simulink model "simple_PD"  (R2021a)
settings: Solver=FixedStepAuto  StartTime=0.0  StopTime=inf  FixedStep=.001  RelTol=1e-3  EnableMultiTasking=on
model workspace (MAT data in the model file):
  SL_ROS_VariableLengthArrays_MaxSizes.CommonInfo.ArrayTruncateAction = 'EmitWarning'
  SL_ROS_VariableLengthArrays_MaxSizes.MsgTypeMap = containers.Map
  SL_ROS_VariableLengthArrays_MaxSizes.MsgTypeMap.serialization.keys = {'ambf_walker/DesiredJoints', 'sensor_msgs/JointState', 'std_msgs/Float32MultiArray'}
  SL_ROS_VariableLengthArrays_MaxSizes.MsgTypeMap.serialization.values{1}(1).PropertyName = 'Controller'
  SL_ROS_VariableLengthArrays_MaxSizes.MsgTypeMap.serialization.values{1}(1).DataType = 'uint8'
  SL_ROS_VariableLengthArrays_MaxSizes.MsgTypeMap.serialization.values{1}(1).MaxLength = 8
  SL_ROS_VariableLengthArrays_MaxSizes.MsgTypeMap.serialization.values{1}(2).PropertyName = 'Other'
  SL_ROS_VariableLengthArrays_MaxSizes.MsgTypeMap.serialization.values{1}(2).DataType = 'double'
  SL_ROS_VariableLengthArrays_MaxSizes.MsgTypeMap.serialization.values{1}(2).MaxLength = 7
  SL_ROS_VariableLengthArrays_MaxSizes.MsgTypeMap.serialization.values{1}(3).PropertyName = 'Q'
  SL_ROS_VariableLengthArrays_MaxSizes.MsgTypeMap.serialization.values{1}(3).DataType = 'double'
  SL_ROS_VariableLengthArrays_MaxSizes.MsgTypeMap.serialization.values{1}(3).MaxLength = 7
  SL_ROS_VariableLengthArrays_MaxSizes.MsgTypeMap.serialization.values{1}(4).PropertyName = 'Qd'
  SL_ROS_VariableLengthArrays_MaxSizes.MsgTypeMap.serialization.values{1}(4).DataType = 'double'
  SL_ROS_VariableLengthArrays_MaxSizes.MsgTypeMap.serialization.values{1}(4).MaxLength = 7
  SL_ROS_VariableLengthArrays_MaxSizes.MsgTypeMap.serialization.values{1}(5).PropertyName = 'Qdd'
  SL_ROS_VariableLengthArrays_MaxSizes.MsgTypeMap.serialization.values{1}(5).DataType = 'double'
  SL_ROS_VariableLengthArrays_MaxSizes.MsgTypeMap.serialization.values{1}(5).MaxLength = 7
  SL_ROS_VariableLengthArrays_MaxSizes.MsgTypeMap.serialization.values{2}(1).PropertyName = 'Effort'
  SL_ROS_VariableLengthArrays_MaxSizes.MsgTypeMap.serialization.values{2}(1).DataType = 'double'
  SL_ROS_VariableLengthArrays_MaxSizes.MsgTypeMap.serialization.values{2}(1).MaxLength = 7
  SL_ROS_VariableLengthArrays_MaxSizes.MsgTypeMap.serialization.values{2}(2).PropertyName = 'Name'
  SL_ROS_VariableLengthArrays_MaxSizes.MsgTypeMap.serialization.values{2}(2).DataType = 'std_msgs/String'
  SL_ROS_VariableLengthArrays_MaxSizes.MsgTypeMap.serialization.values{2}(2).MaxLength = 16
  SL_ROS_VariableLengthArrays_MaxSizes.MsgTypeMap.serialization.values{2}(3).PropertyName = 'Position'
  SL_ROS_VariableLengthArrays_MaxSizes.MsgTypeMap.serialization.values{2}(3).DataType = 'double'
  SL_ROS_VariableLengthArrays_MaxSizes.MsgTypeMap.serialization.values{2}(3).MaxLength = 7
  SL_ROS_VariableLengthArrays_MaxSizes.MsgTypeMap.serialization.values{2}(4).PropertyName = 'Velocity'
  SL_ROS_VariableLengthArrays_MaxSizes.MsgTypeMap.serialization.values{2}(4).DataType = 'double'
  SL_ROS_VariableLengthArrays_MaxSizes.MsgTypeMap.serialization.values{2}(4).MaxLength = 7
  SL_ROS_VariableLengthArrays_MaxSizes.MsgTypeMap.serialization.values{3}.PropertyName = 'Data'
  SL_ROS_VariableLengthArrays_MaxSizes.MsgTypeMap.serialization.values{3}.DataType = 'single'
  SL_ROS_VariableLengthArrays_MaxSizes.MsgTypeMap.serialization.values{3}.MaxLength = 7
  SL_ROS_VariableLengthArrays_MaxSizes.MsgTypeMap.serialization.uniformity = 0
  SL_ROS_VariableLengthArrays_MaxSizes.MsgTypeMap.serialization.keyType = 'char'
  SL_ROS_VariableLengthArrays_MaxSizes.MsgTypeMap.serialization.valueType = 'any'
values from neighbouring files (symbols this model uses):
  Dm1 = [Dm_hip, 0.0, 0.0, 0.0, 0.0, 0.0,0 ... (first row only)    [init_PD_Controller.m]
  Km1 = [Km_hip, 0.0, 0.0, 0.0, 0.0, 0.0,0 ... (first row only)    [init_PD_Controller.m]
undefined symbols (not defined in the file or in its folder): Effort, Header, l, mh, Position, Velocity
libraries: robotlib x13
settings Model: Creator=nathanielgoldfarb  LastModifiedBy=nathanielgoldfarb
settings OptimizationCC: StrengthReduction=on  PassReuseOutputArgsAs=Individual arguments  ZeroExternalMemoryAtStartup=off  ZeroInternalMemoryAtStartup=off  MaxStackSize=64  OptimizeBlockOrder=speed  OptimizationPriority=Speed  OptimizationCustomize=off  MultiThreadedLoops=on  EfficientTunableParamExpr=on
settings DebuggingCC: ParameterTunabilityLossMsg=error
settings HardwareCC: ProdBitPerPointer=32  ProdBitPerSizeT=32  ProdBitPerPtrDiffT=32  ProdLargestAtomicFloat=None  ProdIntDivRoundTo=Undefined  ProdEndianess=Unspecified  ProdWordSize=32  ProdHWDeviceType=Generic->Unspecified (assume 32-bit Generic)
settings SFSimCC: MATLABDynamicMemAlloc=off
settings RTWCC: SystemTargetFile=ert.tlc  HardwareBoard=Robot Operating System (ROS)  TLCOptions="-aInlineSetEventsForThisBaseRateFcn=TLC_FALSE -aSuppressMultiTaskScheduler=TLC_FALSE  -aRateBasedStepFcn=0"  TemplateMakefile=ert_default_tmf  Toolchain=Catkin  TargetLang=C++
settings CodeAppCC: ForceParamTrailComments=on  IgnoreCustomStorageClasses=off  OperatorAnnotations=on  SimulinkDataObjDesc=on  SFDataObjDesc=on  InsertBlockDesc=on

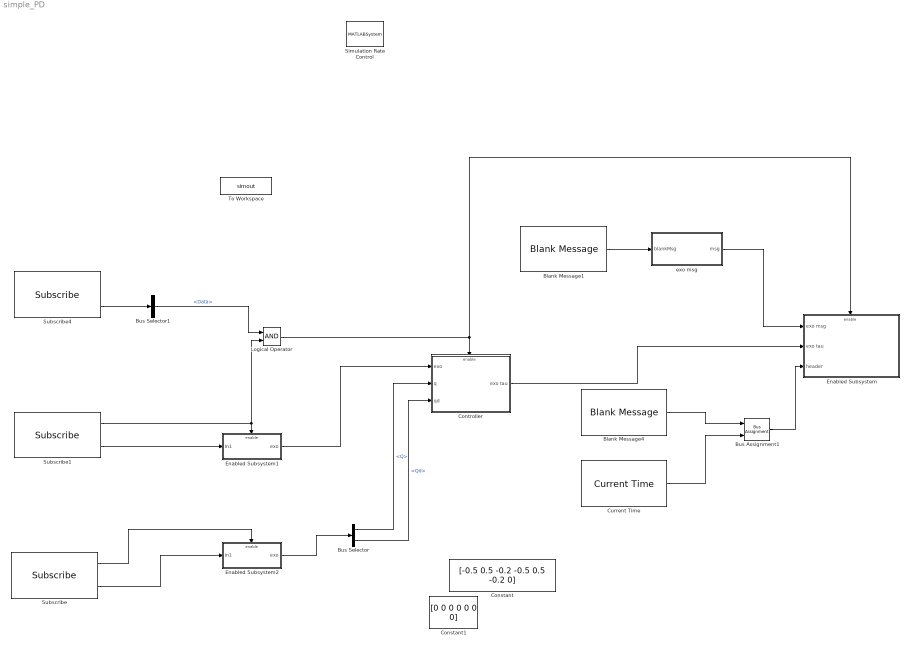
== system simple_PD ==
  Blank Message1 : robotlib/Blank Message  messageClass=Message  entityType=sensor_msgs/JointState  messageType=sensor_msgs/JointState  SampleTime=inf  legacyBusStruct=off
  Blank Message4 : robotlib/Blank Message  messageClass=Message  entityType=std_msgs/Header  messageType=std_msgs/Header  SampleTime=inf  legacyBusStruct=off
  Bus Assignment1 : BusAssignment  AssignedSignals=Stamp
  Bus Selector : BusSelector  OutputSignals=Q,Qd
  Bus Selector1 : BusSelector  OutputSignals=Data
  Constant : Constant  Value=[-0.5 0.5 -0.2 -0.5 0.5 -0.2 0]
  Constant1 : Constant  Value=[0 0 0 0 0 0 0]
  Controller : Subsystem  TreatAsAtomicUnit=on
  Current Time : robotlib/Current Time  OutputFormat=bus  SampleTime=-1  ModelName=simple_PD
      settings: SourceProductBaseCode=RR
  Enabled Subsystem : Subsystem  TreatAsAtomicUnit=on
  Enabled Subsystem1 : Subsystem  TreatAsAtomicUnit=on
  Enabled Subsystem2 : Subsystem  TreatAsAtomicUnit=on
  Logical Operator : Logic  AllPortsSameDT=off  OutDataTypeStr=boolean
  Simulation Rate Control : MATLABSystem  System=ExampleHelperSimulationRateControl  SampleTime=0.001
      mask Type: ExampleHelperSimulationRateControl
      mask Display:
      | disp('Rate Control');
      | port_label('output',1,'r');
  Subscribe : robotlib/Subscribe  topicSource=Select from ROS network  topic=/exosimulink_set_points  messageType=ambf_walker/DesiredJoints  SampleTime=-1  legacyBusStruct=off  messageQueueLength=1
  Subscribe1 : robotlib/Subscribe  topicSource=Select from ROS network  topic=/exo_jointstate  messageType=sensor_msgs/JointState  SampleTime=-1  legacyBusStruct=off  messageQueueLength=1
  Subscribe4 : robotlib/Subscribe  topicSource=Specify your own  topic=/start_sim  messageType=std_msgs/Bool  SampleTime=-1  legacyBusStruct=off  messageQueueLength=1
  To Workspace : ToWorkspace  VariableName=simout  SampleTime=-1
      settings: Save2DSignal=2-D array (concatenate along first dimension)
  exo msg : MATLAB Function  TreatAsAtomicUnit=on
  wires:
  Bus Assignment1/1 -> Enabled Subsystem/3(header)
  Blank Message1/1 -> exo msg/1(blankMsg)
  exo msg/1(msg) -> Enabled Subsystem/1(exo msg)
  Current Time/1 -> Bus Assignment1/2
  Blank Message4/1 -> Bus Assignment1/1
  Enabled Subsystem1/1(exo) -> Controller/1(exo)
  Subscribe4/2 -> Bus Selector1/1
  Subscribe1/2 -> Enabled Subsystem1/1(In1)
  Controller/1(exo tau) -> Enabled Subsystem/2(exo tau)
  Subscribe1/1 -> Enabled Subsystem1/Enable, Logical Operator/2
  Subscribe/2 -> Enabled Subsystem2/1(In1)
  Enabled Subsystem2/1(exo) -> Bus Selector/1
  Subscribe/1 -> Enabled Subsystem2/Enable
  Bus Selector1/1 -> Logical Operator/1  "<Data>"
  Logical Operator/1 -> Enabled Subsystem/Enable, Controller/Enable
  Bus Selector/1 -> Controller/2(q)  "<Q>"
  Bus Selector/2 -> Controller/3(qd)  "<Qd>"

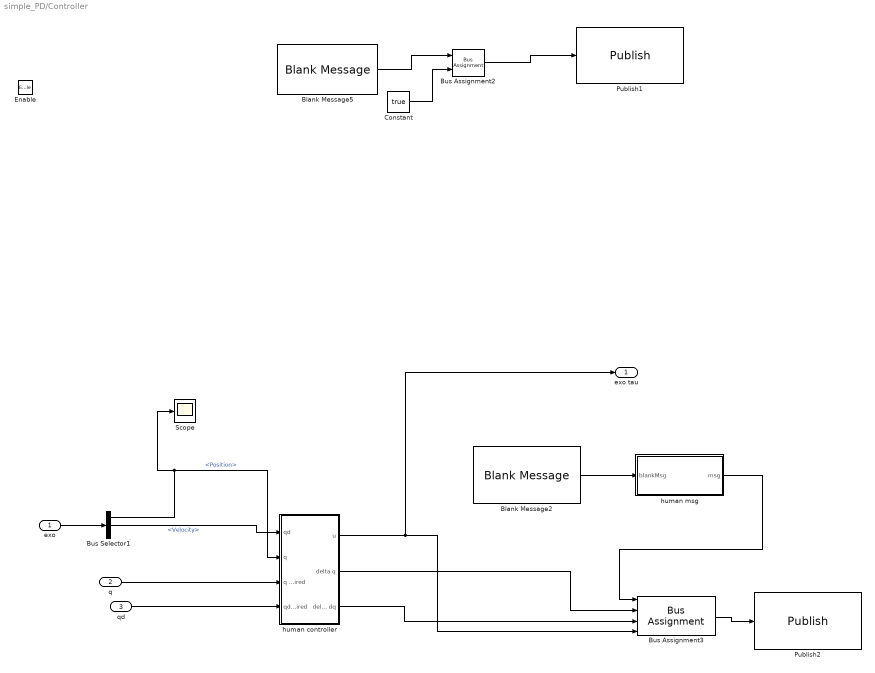
== system simple_PD/Controller ==
  exo : Inport
  q : Inport  Port=2
  qd : Inport  Port=3
  Enable : EnablePort
  Blank Message2 : robotlib/Blank Message  messageClass=Message  entityType=sensor_msgs/JointState  messageType=sensor_msgs/JointState  SampleTime=inf  legacyBusStruct=off
  Blank Message5 : robotlib/Blank Message  messageClass=Message  entityType=std_msgs/Bool  messageType=std_msgs/Bool  SampleTime=inf  legacyBusStruct=off
  Bus Assignment2 : BusAssignment  AssignedSignals=Data
  Bus Assignment3 : BusAssignment  AssignedSignals=Position,Velocity,Effort
  Bus Selector1 : BusSelector  OutputSignals=Position,Velocity,Effort
  Constant : Constant  Value=true  VectorParams1D=off
  Publish1 : robotlib/Publish  topicSource=Specify your own  topic=/my_topic  messageType=std_msgs/Bool  legacyBusStruct=off  messageQueueLength=1
  Publish2 : robotlib/Publish  topicSource=Specify your own  topic=addmittance  messageType=sensor_msgs/JointState  legacyBusStruct=off  messageQueueLength=1
  Scope : Scope
  human controller : Subsystem
  human msg : MATLAB Function  TreatAsAtomicUnit=on
  exo tau : Outport
  wires:
  q/1 -> human controller/3(q desired)
  qd/1 -> human controller/4(qd desired)
  Bus Selector1/1 -> human controller/2(q), Scope/1  "<Position>"
  exo/1 -> Bus Selector1/1
  Constant/1 -> Bus Assignment2/2
  Blank Message5/1 -> Bus Assignment2/1
  Bus Assignment2/1 -> Publish1/1
  Bus Assignment3/1 -> Publish2/1
  Blank Message2/1 -> human msg/1(blankMsg)
  human msg/1(msg) -> Bus Assignment3/1
  Bus Selector1/2 -> human controller/1(qd)  "<Velocity>"
  human controller/2(delta q) -> Bus Assignment3/2
  human controller/3(delta dq) -> Bus Assignment3/3
  human controller/1(u) -> exo tau/1, Bus Assignment3/4

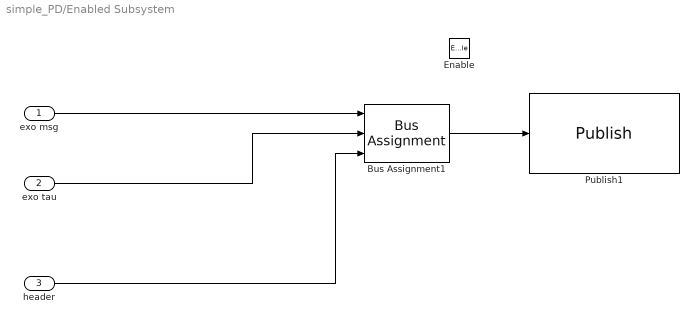
== system simple_PD/Enabled Subsystem ==
  exo msg : Inport
  exo tau : Inport  Port=2
  header : Inport  Port=3
  Enable : EnablePort
  Bus Assignment1 : BusAssignment  AssignedSignals=Effort,Header
  Publish1 : robotlib/Publish  topicSource=Select from ROS network  topic=/exo_simulink_torque  messageType=sensor_msgs/JointState  legacyBusStruct=off  messageQueueLength=1
  wires:
  exo tau/1 -> Bus Assignment1/2
  Bus Assignment1/1 -> Publish1/1
  exo msg/1 -> Bus Assignment1/1
  header/1 -> Bus Assignment1/3

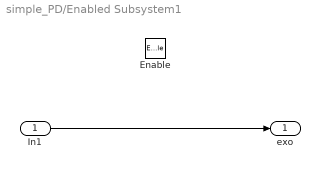
== system simple_PD/Enabled Subsystem1 ==
  In1 : Inport
  Enable : EnablePort
  exo : Outport
  wires:
  In1/1 -> exo/1

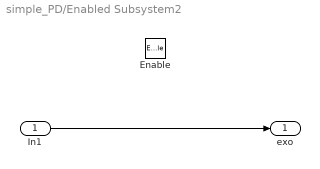
== system simple_PD/Enabled Subsystem2 ==
  In1 : Inport
  Enable : EnablePort
  exo : Outport
  wires:
  In1/1 -> exo/1

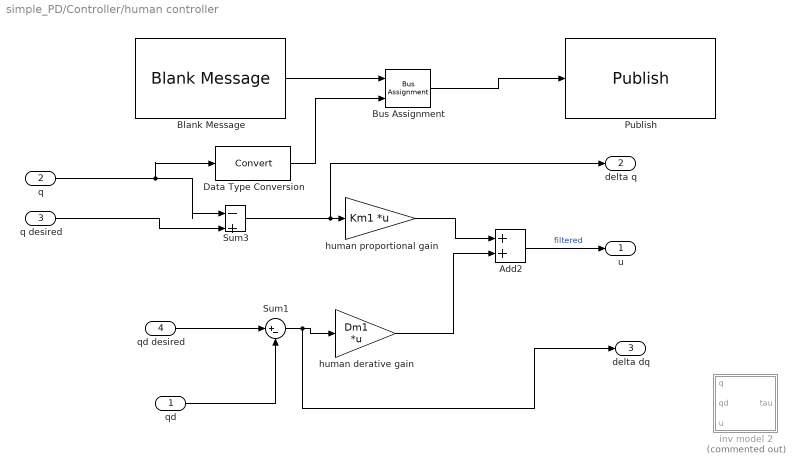
== system simple_PD/Controller/human controller ==
  qd : Inport
  q : Inport  Port=2
  q desired : Inport  Port=3
  qd desired : Inport  Port=4
  Add2 : Sum
  Blank Message : robotlib/Blank Message  messageClass=Message  entityType=std_msgs/Float32MultiArray  messageType=std_msgs/Float32MultiArray  SampleTime=inf  legacyBusStruct=off
  Bus Assignment : BusAssignment  AssignedSignals=Data
  Data Type Conversion : DataTypeConversion  RndMeth=Simplest
  Publish : robotlib/Publish  topicSource=Specify your own  topic=PD_error  messageType=std_msgs/Float32MultiArray  legacyBusStruct=off  messageQueueLength=1
  Sum1 : Sum  Inputs=|+-
  Sum3 : Sum  Inputs=|-+
  human derative gain : Gain  Gain=Dm1  Multiplication=Matrix(K*u)
  human proportional gain : Gain  Gain=Km1  Multiplication=Matrix(K*u)
  inv model 2 : Subsystem  Commented=on
  u : Outport
  delta q : Outport  Port=2
  delta dq : Outport  Port=3
  wires:
  Sum1/1 -> delta dq/1, human derative gain/1
  qd/1 -> Sum1/2
  Sum3/1 -> delta q/1, human proportional gain/1
  human derative gain/1 -> Add2/2
  q desired/1 -> Sum3/2
  human proportional gain/1 -> Add2/1
  qd desired/1 -> Sum1/1
  q/1 -> Data Type Conversion/1, Sum3/1
  Add2/1 -> u/1  "filtered"
  Blank Message/1 -> Bus Assignment/1
  Bus Assignment/1 -> Publish/1
  Data Type Conversion/1 -> Bus Assignment/2

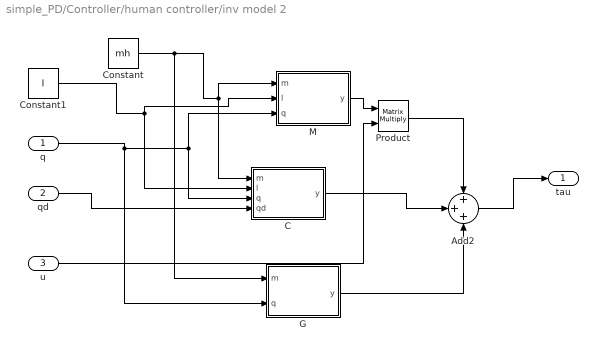
== system simple_PD/Controller/human controller/inv model 2 ==
  q : Inport
  qd : Inport  Port=2
  "u " : Inport  Port=3
  Add2 : Sum  Inputs=+++
  C : MATLAB Function  TreatAsAtomicUnit=on
  Constant : Constant  Value=mh
  Constant1 : Constant  Value=l
  G : MATLAB Function  TreatAsAtomicUnit=on
  M : MATLAB Function  TreatAsAtomicUnit=on
  Product : Product  Multiplication=Matrix(*)
  "tau " : Outport
  wires:
  Constant1/1 -> C/2(l), M/2(l)
  Constant/1 -> G/1(m), C/1(m), M/1(m)
  "u "/1 -> Product/2
  Product/1 -> Add2/1
  M/1(y) -> Product/1
  qd/1 -> C/4(qd)
  q/1 -> G/2(q), C/3(q), M/3(q)
  Add2/1 -> "tau "/1
  C/1(y) -> Add2/2
  G/1(y) -> Add2/3

== matlab function simple_PD/Controller/human controller/inv model 2/C ==
  data: m input; l input; q input; y output; qd input
function y = fcn(m, l, q, qd)



y = C(m, l, q, qd); % [m(2)*l(2)*qd(2)*qd(2)*sin(q(1)-q(2)); -m(2)*l(1)*qd(1)*qd(1)*sin(q(1)-q(2))];

== matlab function simple_PD/Controller/human controller/inv model 2/G ==
  data: m input; q input; y output
function y = fcn(m, q)
 y =  G(m,q);
end

== matlab function simple_PD/Controller/human controller/inv model 2/M ==
  data: m input; l input; q input; y output
function y = fcn(m, l, q)

y = M(m,l,q); % pinv([ (m(1)+m(2)) *l(1), m(2)*l(2)*cos(q(1)-q(2)); m(2)* l(1)*cos(q(1)-q(2)), m(2)*l(2)] );

end

== matlab function simple_PD/exo msg ==
  data: blankMsg input; msg output Bus: SL_Bus_simple_PD_sensor_msgs_JointState
function msg = stringArrayAssign(blankMsg)
% stringArrayAssign - Assign a string array in a ROS message
%
%  blankMsg (input): A bus for a 'sensor_msgs/JointState' message. This is 
%      used to initialize the output.
%  msg (output): A bus for a 'sensor_msgs/JointState' message message, with 
%      Name field set to a string array.
%
%   Copyright 2015 The MathWorks, Inc.

%#codegen

% Note: The datatype of 'msg' has been explicitly set to the appropriate 
% Simulink bus type ("SL_Bus_robotROSMessageUsageExample_sensor_msgs_JointState"). 
%
% If the model name is changed, the datatype needs to be changed as well:
%   1) Click "Edit Data" in the Editor toolstrip to open "Ports and Data Manager"
%   2) Select "msg". From the "Type" dropdown, select "--- Refresh data types ---"
%   3) Set datatype to "Bus: SL_Bus_<modelname>_sensor_msgs_JointState"

strArrayToAssign = {'LeftExoHip', 'LeftExoKnee', 'LeftExoAnkle', 'RightExoHip', 'RightExoKnee', 'RightExoAnkle', 'Crutches'};
msg = blankMsg;

% Set the number of strings in the string array.
% msg (sensor_msgs/JointState) includes the following fields
%           Name : array of std_msgs/String (string array)
%   Name_SL_Info : struct with fields CurrentLength, ReceivedLength
numStringsInArray = length(strArrayToAssign);
msg.Name_SL_Info.CurrentLength = uint32(numStringsInArray);
msg.Effort_SL_Info.CurrentLength = uint32(numStringsInArray);

% Set the individual strings in the array
for idx=1:numStringsInArray
    str = strArrayToAssign{idx};
    strLength = length(str);
    msg.Name(idx).Data(1:strLength) = uint8(str);
    msg.Name(idx).Data_SL_Info.CurrentLength = uint32(strLength);
end

== matlab function simple_PD/Controller/human msg ==
  data: blankMsg input; msg output Bus: SL_Bus_simple_PD_sensor_msgs_JointState
function msg = stringArrayAssign(blankMsg)
% stringArrayAssign - Assign a string array in a ROS message
%
%  blankMsg (input): A bus for a 'sensor_msgs/JointState' message. This is 
%      used to initialize the output.
%  msg (output): A bus for a 'sensor_msgs/JointState' message message, with 
%      Name field set to a string array.
%
%   Copyright 2015 The MathWorks, Inc.

%#codegen

% Note: The datatype of 'msg' has been explicitly set to the appropriate 
% Simulink bus type ("SL_Bus_robotROSMessageUsageExample_sensor_msgs_JointState"). 
%
% If the model name is changed, the datatype needs to be changed as well:
%   1) Click "Edit Data" in the Editor toolstrip to open "Ports and Data Manager"
%   2) Select "msg". From the "Type" dropdown, select "--- Refresh data types ---"
%   3) Set datatype to "Bus: SL_Bus_<modelname>_sensor_msgs_JointState"

strArrayToAssign = {'LeftHip', 'LeftKnee', 'LeftAnkle', 'RightHip', 'RightKnee', 'RightAnkle', 'blanck'};
msg = blankMsg;

% Set the number of strings in the string array.
% msg (sensor_msgs/JointState) includes the following fields
%           Name : array of std_msgs/String (string array)
%   Name_SL_Info : struct with fields CurrentLength, ReceivedLength
numStringsInArray = length(strArrayToAssign);
msg.Name_SL_Info.CurrentLength = uint32(numStringsInArray);
msg.Velocity_SL_Info.CurrentLength = uint32(numStringsInArray);
msg.Position_SL_Info.CurrentLength = uint32(numStringsInArray);
msg.Effort_SL_Info.CurrentLength = uint32(numStringsInArray);

% Set the individual strings in the array
for idx=1:numStringsInArray
    str = strArrayToAssign{idx};
    strLength = length(str);
    msg.Name(idx).Data(1:strLength) = uint8(str);
    msg.Name(idx).Data_SL_Info.CurrentLength = uint32(strLength);
end
